simulink model "team_model_v1.2"  (R2022a)
settings: Solver=VariableStepAuto  StartTime=0.0  StopTime=10.0  RelTol=1e-3
undefined symbols (not defined in the file): dfilt, DiscIntNeverNeededParam, sigbuilder_block
libraries: visionsources x8, simulink x6, dsparch4 x5, dspvision x3, audioeffects x2, dspsnks4 x1, commanapbnd3 x1, commsynccomp2 x1
settings Model: Creator=Yogesh  LastModifiedBy=loges

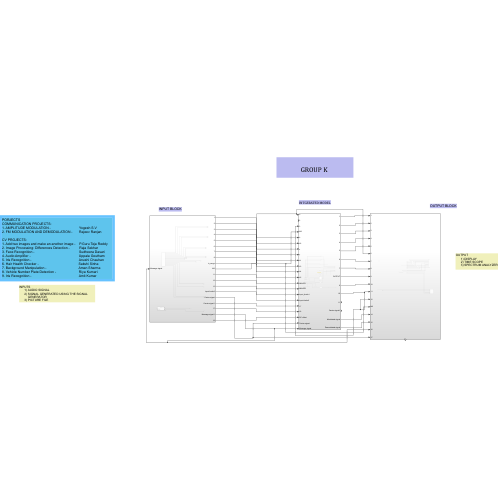
[thumbnail: Simulink's stored preview of the top-level diagram]
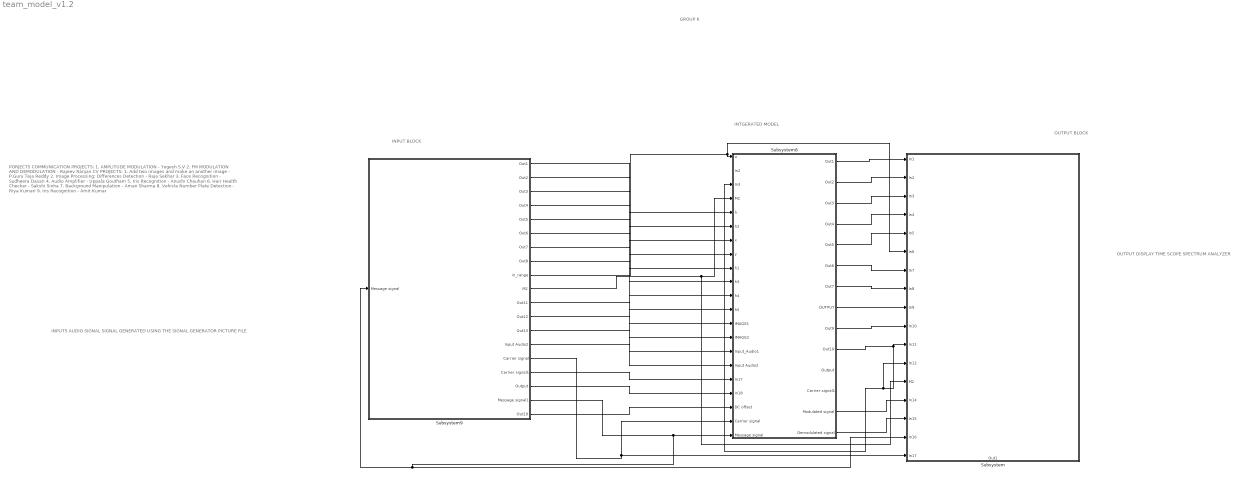
== system team_model_v1.2 ==
  note: OUTPUT
      | DISPLAY
      | TIME SCOPE
      | SPECTRUM ANALYZER
  note: INPUTS
      | AUDIO SIGNAL
      | SIGNAL GENERATED USING THE SIGNAL GENERATOR
      | PICTURE FILE
  note: PORJECTS
      | COMMUNICATION PROJECTS:
      | 1. AMPLITUDE MODULATION - Yogesh S.V
      | 2. FM MODULATION AND DEMODULATION - Rajeev Ranjan
      |
      | CV PROJECTS:
      | 1. Add two images and make an another image - P.Guru Teja Reddy
      | 2. Image Processing: Differences Detection - Raja Sekhar
      | 3. Face Recognition - Sudheera Dasari
      | 4. Audio Amplifier - Uppala Goutham
      | 5. Iris Recognition - Anushi Chauhan
      | 6. Hair Health Checker - Sakshi Sinha
      | 7. Background Manipulation - Aman Sharma
      | 8. Vehicle Number Plate Detection - Riya Kumari
      | 9. Iris Recognition - Amit Kumar
  note: GROUP K
  note: OUTPUT BLOCK
  note: INPUT BLOCK
  note: INTGERATED MODEL
  Subsystem : Subsystem
      settings: PortSchema="{\"entries\":[{\"content\":{\"sides\":[{\"content\":{\"connectorIds\":[\"In1\",\"In2\",\"In3\",\"In4\",\"In5\",\"In6\",\"In7\",\"In8\",\"In9\",\"In10\",\"In11\",\"In12\",\"In13\",\"In14\",\"In15\",\"In16\",\"In17\"]},\"type\":\"ConnectorPlacement.EquallySpacedRectSide\",\"uuid\":\"30eb3b3b-e642-47c5-bd95-9ad21aad3d43\"},{\"content\":{\"connectorIds\":[],\"side\":\"RIGHT\"},\"type\":\"ConnectorPlacement.EquallySpacedRectSide\",\"uuid\":\"7c869e27-b9a3-4d84-b0f1-035dc5e7d885\"},{\"content\":{\"connectorIds\":[],\"side\":\"TOP\"},\"type\":\"ConnectorPlacement.EquallySpacedRectSide\",\"uuid\":\"1cca7824-1698-4971-845e-a337e380de9b\"},{\"content\":{\"connectorIds\":[\"Out1\"],\"side\":\"BOTTOM\"},\"type\":\"ConnectorPlacement.EquallySpacedRectSide\",\"uuid\":\"e608f006-b2e8-4151-859e-ece5e69022af\"}]},\"type\":\"ConnectorPlacement.EquallySpacedConnector\",\"uuid\":\"a6df2039-72ad-42ba-adc3-335df7237120\"}],\"packageUris\":[\"http://schema.mathworks.com/mf0/Connector/R2020b\"],\"version\":\"1.0\"}"
  Subsystem8 : Subsystem
  Subsystem9 : Subsystem
  wires:
  Subsystem9/9(in_range) -> Subsystem8/1(u), Subsystem/6(In6)
  Subsystem9/10(M2) -> Subsystem/13(M2), Subsystem8/4(M2)
  Subsystem9/15(Carrier signal) -> Subsystem8/20(Carrier signal), Subsystem/17(In17)
  Subsystem9/18(Message signal1) -> Subsystem/16(In16), Subsystem9/1(Message signal), Subsystem8/21(Message signal)
  Subsystem8/10(Out10) -> Subsystem8/3(In3), Subsystem/12(In12), Subsystem/11(In11)
  Subsystem9/1(Out1) -> Subsystem8/5(h)
  Subsystem9/2(Out2) -> Subsystem8/6(h2)
  Subsystem9/3(Out3) -> Subsystem8/7(x)
  Subsystem9/4(Out4) -> Subsystem8/8(y)
  Subsystem9/5(Out5) -> Subsystem8/9(h1)
  Subsystem9/6(Out6) -> Subsystem8/10(h3)
  Subsystem9/7(Out7) -> Subsystem8/11(h4)
  Subsystem9/8(Out8) -> Subsystem8/12(h5)
  Subsystem9/11(Out11) -> Subsystem8/13(IMAGE1)
  Subsystem9/12(Out12) -> Subsystem8/14(IMAGE2)
  Subsystem9/13(Out13) -> Subsystem8/15(Input_Audio1)
  Subsystem9/14(Input Audio2) -> Subsystem8/16(Input Audio2)
  Subsystem9/16(Carrier signal1) -> Subsystem8/17(In17)
  Subsystem9/17(Output) -> Subsystem8/18(In18)
  Subsystem9/19(Out19) -> Subsystem8/19(DC offset)
  Subsystem8/1(Out1) -> Subsystem/1(In1)
  Subsystem8/2(Out2) -> Subsystem/2(In2)
  Subsystem8/3(Out3) -> Subsystem/3(In3)
  Subsystem8/4(Out4) -> Subsystem/4(In4)
  Subsystem8/5(Out5) -> Subsystem/5(In5)
  Subsystem8/6(Out6) -> Subsystem/7(In7)
  Subsystem8/7(Out7) -> Subsystem/8(In8)
  Subsystem8/8(OUTPUT) -> Subsystem/9(In9)
  Subsystem8/9(Out9) -> Subsystem/10(In10)
  Subsystem8/13(Modulated signal) -> Subsystem/14(In14)
  Subsystem8/14(Demodulated signal) -> Subsystem/15(In15)

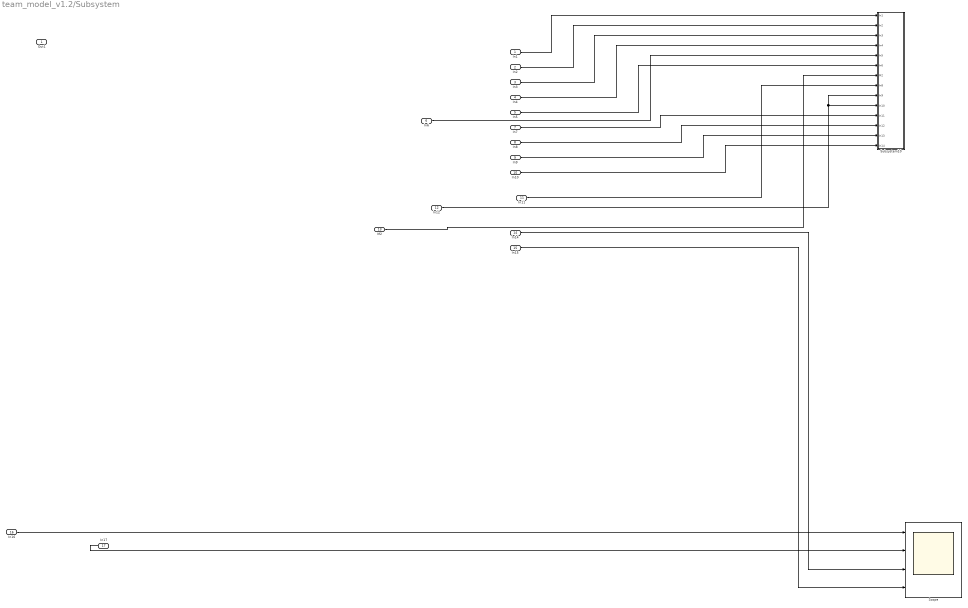
== system team_model_v1.2/Subsystem ==
  In1 : Inport
  In2 : Inport  Port=2
  In3 : Inport  Port=3
  In4 : Inport  Port=4
  In5 : Inport  Port=5
  In6 : Inport  Port=6
  In7 : Inport  Port=7
  In8 : Inport  Port=8
  In9 : Inport  Port=9
  In10 : Inport  Port=10
  In11 : Inport  Port=11
  In12 : Inport  Port=12
  M2 : Inport  Port=13
  In14 : Inport  Port=14
  In15 : Inport  Port=15
  In16 : Inport  Port=16
  In17 : Inport  Port=17
  Scope : Scope  NumInputPorts=4
  Subsystem10 : Subsystem
  Out1 : Outport
  wires:
  In16/1 -> Scope/1
  In12/1 -> Subsystem10/9(In9), Subsystem10/10(In10)
  In4/1 -> Subsystem10/4(In4)
  In10/1 -> Subsystem10/14(In14)
  In3/1 -> Subsystem10/3(In3)
  In11/1 -> Subsystem10/8(In8)
  In5/1 -> Subsystem10/6(In6)
  In2/1 -> Subsystem10/2(In2)
  In1/1 -> Subsystem10/1(In1)
  In6/1 -> Subsystem10/5(In5)
  In8/1 -> Subsystem10/12(In12)
  In7/1 -> Subsystem10/11(In11)
  In9/1 -> Subsystem10/13(In13)
  M2/1 -> Subsystem10/7(M2)
  In14/1 -> Scope/3
  In17/1 -> Scope/2
  In15/1 -> Scope/4

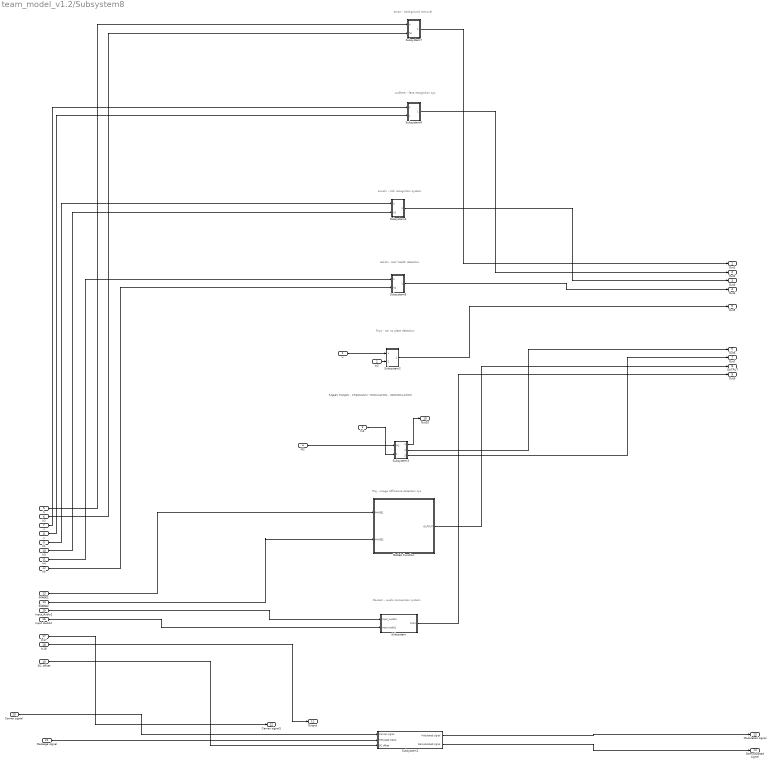
== system team_model_v1.2/Subsystem8 ==
  note: sudhera - face recognition sys
  note: anushi - irish recognition system
  note: sakshi - Hair health detection
  note: Riya - car no plate detection
  note: Raj - image difference detection sys
  note: Goutam - audio comaprison system
  note: RAJEEV RANJAN - FREQUENCY MODULATION - DEMODULATION
  note: Aman - background removal
  u : Inport
  In2 : Inport  Port=2
  In3 : Inport  Port=3
  M2 : Inport  Port=4
  h : Inport  Port=5
  h2 : Inport  Port=6
  x : Inport  Port=7
  y : Inport  Port=8
  h1 : Inport  Port=9
  h3 : Inport  Port=10
  h4 : Inport  Port=11
  h5 : Inport  Port=12
  IMAGE1 : Inport  Port=13
  IMAGE2 : Inport  Port=14
  Input_Audio1 : Inport  Port=15
  Input Audio2 : Inport  Port=16
  In17 : Inport  Port=17
  In18 : Inport  Port=18
  DC offset : Inport  Port=19
  Carrier signal : Inport  Port=20
  Message signal : Inport  Port=21
  Matlab Function : Subsystem
  Subsystem : Subsystem
  Subsystem1 : Subsystem
  Subsystem2 : Subsystem
  Subsystem3 : Subsystem
  Subsystem4 : Subsystem
  Subsystem5 : Subsystem
  Subsystem6 : Subsystem
  Subsystem7 : Subsystem
  Out1 : Outport
  Out2 : Outport  Port=2
  Out3 : Outport  Port=3
  Out4 : Outport  Port=4
  Out5 : Outport  Port=5
  Out6 : Outport  Port=6
  Out7 : Outport  Port=7
  OUTPUT : Outport  Port=8
  Out9 : Outport  Port=9
  Out10 : Outport  Port=10
  Output : Outport  Port=11
  Carrier signal1 : Outport  Port=12
  Modulated signal : Outport  Port=13
  Demodulated signal : Outport  Port=14
  wires:
  M2/1 -> Subsystem3/1(M2)
  Subsystem6/1(Out1) -> Out2/1
  Subsystem2/1(Out1) -> Out5/1
  y/1 -> Subsystem6/2(y)
  Subsystem3/2(Out2) -> Out6/1
  Subsystem7/1(Out1) -> Out1/1
  Subsystem3/3(Out3) -> Out7/1
  Subsystem5/1(Out1) -> Out4/1
  h3/1 -> Subsystem4/2(h2)
  Subsystem4/1(Out1) -> Out3/1
  u/1 -> Subsystem2/1(u)
  Matlab Function/1(OUTPUT) -> OUTPUT/1
  Subsystem/1(Out1) -> Out9/1
  h/1 -> Subsystem7/1(h)
  h2/1 -> Subsystem7/2(h2)
  x/1 -> Subsystem6/1(x)
  IMAGE2/1 -> Matlab Function/2(IMAGE2)
  Input_Audio1/1 -> Subsystem/1(Input_Audio1)
  h4/1 -> Subsystem5/1(h)
  In17/1 -> Carrier signal1/1
  Subsystem1/2(Demodulated signal) -> Demodulated signal/1
  IMAGE1/1 -> Matlab Function/1(IMAGE1)
  h1/1 -> Subsystem4/1(h)
  h5/1 -> Subsystem5/2(h2)
  In2/1 -> Subsystem2/2(In2)
  DC offset/1 -> Subsystem1/3(DC offset)
  In18/1 -> Output/1
  Input Audio2/1 -> Subsystem/2(Input Audio2)
  Message signal/1 -> Subsystem1/2(Message signal)
  Subsystem1/1(Modulated signal) -> Modulated signal/1
  Carrier signal/1 -> Subsystem1/1(Carrier signal)
  Subsystem3/1(Out1) -> Out10/1
  In3/1 -> Subsystem3/2(In2)

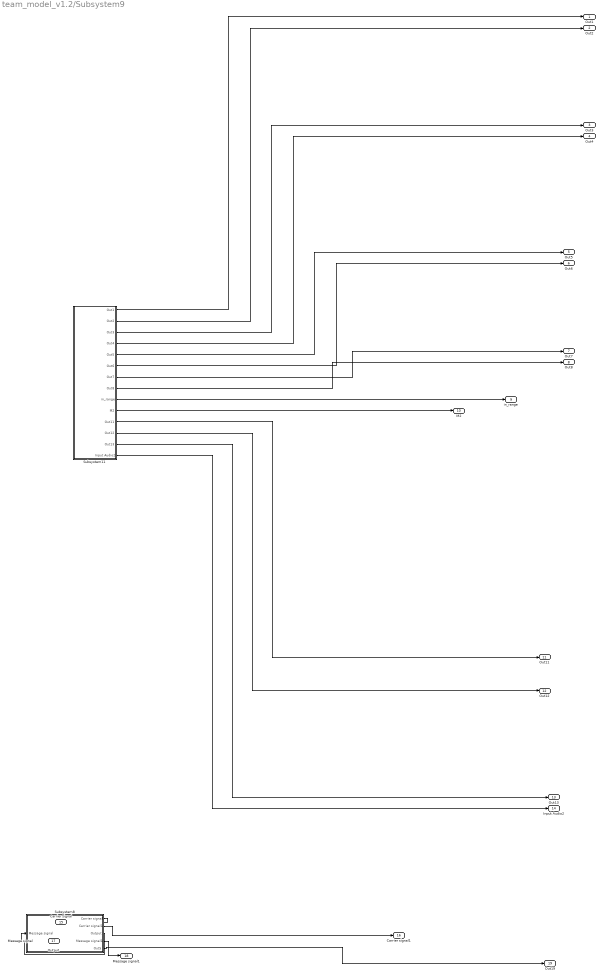
== system team_model_v1.2/Subsystem9 ==
  Message signal : Inport
  Subsystem11 : Subsystem
  Subsystem8 : Subsystem
  Out1 : Outport
  Out2 : Outport  Port=2
  Out3 : Outport  Port=3
  Out4 : Outport  Port=4
  Out5 : Outport  Port=5
  Out6 : Outport  Port=6
  Out7 : Outport  Port=7
  Out8 : Outport  Port=8
  in_range : Outport  Port=9
  M2 : Outport  Port=10
  Out11 : Outport  Port=11
  Out12 : Outport  Port=12
  Out13 : Outport  Port=13
  Input Audio2 : Outport  Port=14
  Carrier signal : Outport  Port=15
  Carrier signal1 : Outport  Port=16
  Output : Outport  Port=17
  Message signal1 : Outport  Port=18
  Out19 : Outport  Port=19
  wires:
  Subsystem8/5(Out5) -> Out19/1
  Subsystem8/3(Output) -> Output/1
  Subsystem8/1(Carrier signal) -> Carrier signal/1
  Subsystem11/2(Out2) -> Out2/1
  Message signal/1 -> Subsystem8/1(Message signal)
  Subsystem8/4(Message signal1) -> Message signal1/1
  Subsystem11/1(Out1) -> Out1/1
  Subsystem8/2(Carrier signal1) -> Carrier signal1/1
  Subsystem11/3(Out3) -> Out3/1
  Subsystem11/5(Out5) -> Out5/1
  Subsystem11/4(Out4) -> Out4/1
  Subsystem11/12(Out12) -> Out12/1
  Subsystem11/13(Out13) -> Out13/1
  Subsystem11/10(M2) -> M2/1
  Subsystem11/9(in_range) -> in_range/1
  Subsystem11/6(Out6) -> Out6/1
  Subsystem11/7(Out7) -> Out7/1
  Subsystem11/11(Out11) -> Out11/1
  Subsystem11/8(Out8) -> Out8/1
  Subsystem11/14(Input Audio2) -> Input Audio2/1

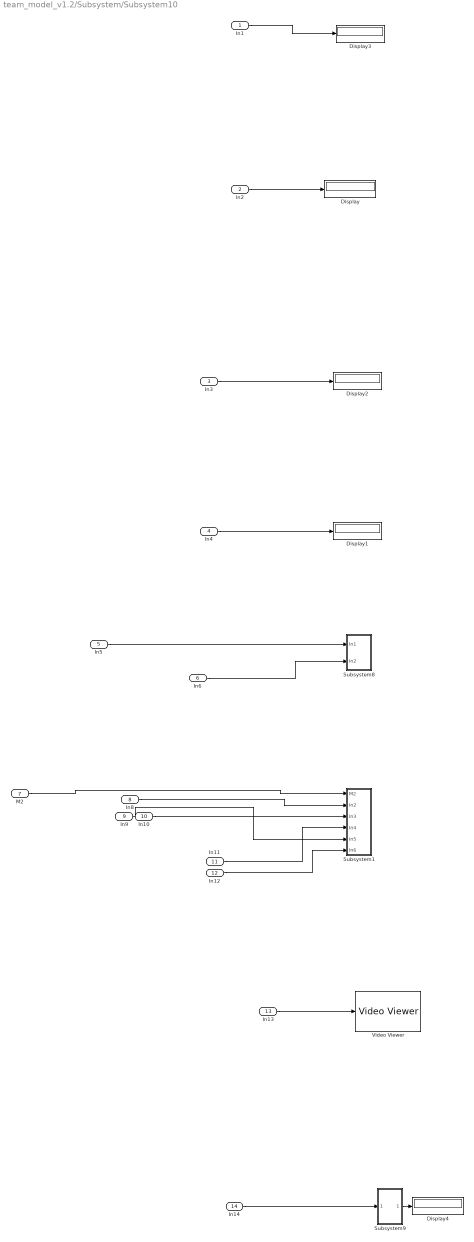
== system team_model_v1.2/Subsystem/Subsystem10 ==
  In1 : Inport
  In2 : Inport  Port=2
  In3 : Inport  Port=3
  In4 : Inport  Port=4
  In5 : Inport  Port=5
  In6 : Inport  Port=6
  M2 : Inport  Port=7
  In8 : Inport  Port=8
  In9 : Inport  Port=9
  In10 : Inport  Port=10
  In11 : Inport  Port=11
  In12 : Inport  Port=12
  In13 : Inport  Port=13
  In14 : Inport  Port=14
  Display{,1..4} (5 alike) : Display
  Subsystem1 : Subsystem
  Subsystem8 : Subsystem
  Subsystem9 : Subsystem
  Video Viewer : VideoViewer  FigPos=[1376 392 357 191]
  wires:
  In3/1 -> Display2/1
  In8/1 -> Subsystem1/2(In2)
  In13/1 -> Video Viewer/1
  In14/1 -> Subsystem9/1(In1)
  In9/1 -> Subsystem1/5(In5)
  In10/1 -> Subsystem1/3(In3)
  In1/1 -> Display3/1
  Subsystem9/1(Out1) -> Display4/1
  In4/1 -> Display1/1
  In2/1 -> Display/1
  In5/1 -> Subsystem8/1(In1)
  In6/1 -> Subsystem8/2(In2)
  In11/1 -> Subsystem1/4(In4)
  M2/1 -> Subsystem1/1(M2)
  In12/1 -> Subsystem1/6(In6)

== system team_model_v1.2/Subsystem8/Matlab Function ==
  IMAGE1 : Inport
  IMAGE2 : Inport  Port=2
  MATLAB Function : MATLAB Function  TreatAsAtomicUnit=on
  OUTPUT : Outport
  wires:
  IMAGE2/1 -> MATLAB Function/2(y)
  IMAGE1/1 -> MATLAB Function/1(x)
  MATLAB Function/1(z) -> OUTPUT/1

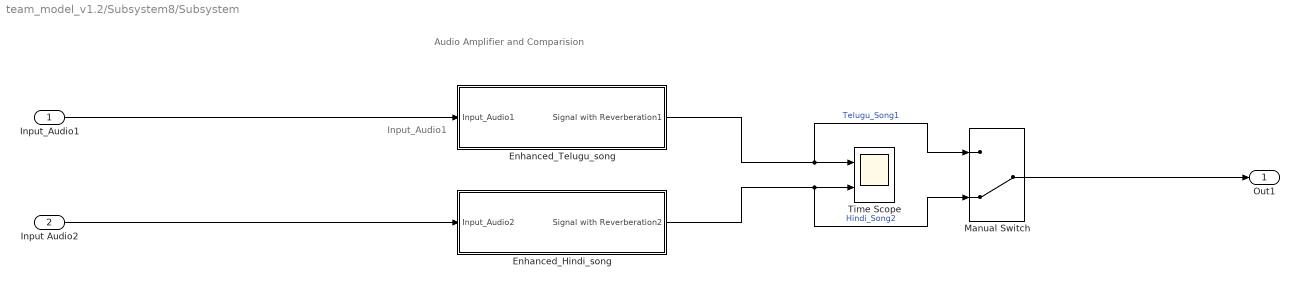
== system team_model_v1.2/Subsystem8/Subsystem ==
  note: Audio Amplifier and Comparision
  note: Input_Audio1
  Input_Audio1 : Inport
  Input Audio2 : Inport  Port=2
  " Manual Switch" : ManualSwitch  CurrentSetting=0
  Enhanced_Hindi_song : Subsystem
  Enhanced_Telugu_song : Subsystem
  Time Scope : Scope  NumInputPorts=2
  Out1 : Outport
  wires:
  " Manual Switch"/1 -> Out1/1
  Enhanced_Hindi_song/1(Signal with Reverberation2) -> " Manual Switch"/2, Time Scope/2  "Hindi_Song2"
  Enhanced_Telugu_song/1(Signal with Reverberation1) -> " Manual Switch"/1, Time Scope/1  "Telugu_Song1"
  Input Audio2/1 -> Enhanced_Hindi_song/1(Input_Audio2)
  Input_Audio1/1 -> Enhanced_Telugu_song/1(Input_Audio1)

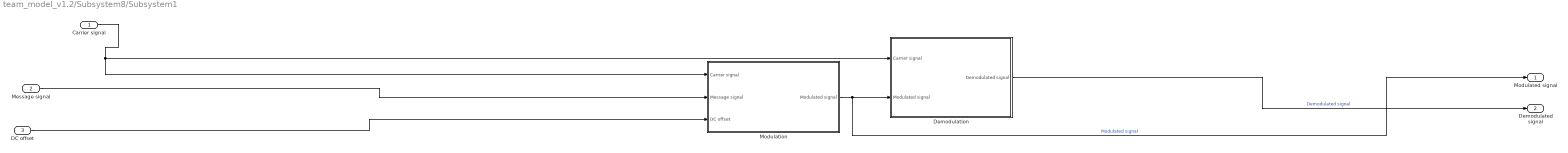
== system team_model_v1.2/Subsystem8/Subsystem1 ==
  Carrier signal : Inport
  Message signal : Inport  Port=2
  DC offset : Inport  Port=3
  Demodulation : Subsystem
  Modulation : Subsystem
  Modulated signal : Outport
  Demodulated signal : Outport  Port=2
  wires:
  Message signal/1 -> Modulation/2(Message signal)
  Modulation/1(Modulated signal) -> Modulated signal/1, Demodulation/2(Modulated signal)  "Modulated signal"
  DC offset/1 -> Modulation/3(DC offset)
  Carrier signal/1 -> Demodulation/1(Carrier signal), Modulation/1(Carrier signal)
  Demodulation/1(Demodulated signal) -> Demodulated signal/1  "Demodulated signal"

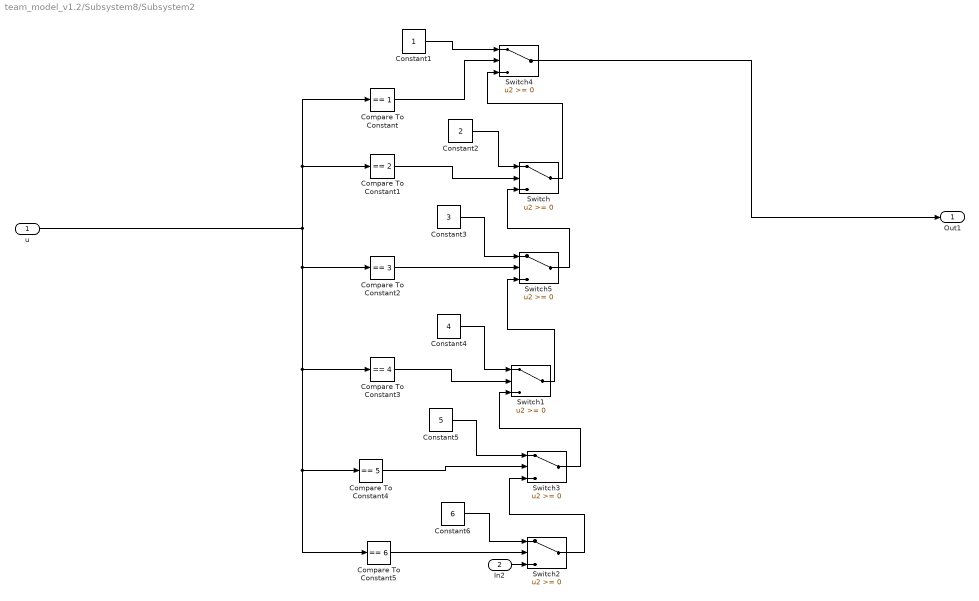
== system team_model_v1.2/Subsystem8/Subsystem2 ==
  u : Inport
  In2 : Inport  Port=2
  Compare To Constant : simulink/Logic and Bit Operations/Compare To Constant  relop===  const=1  OutDataTypeStr=boolean
  Compare To Constant1 : simulink/Logic and Bit Operations/Compare To Constant  relop===  const=2  OutDataTypeStr=boolean
  Compare To Constant2 : simulink/Logic and Bit Operations/Compare To Constant  relop===  const=3  OutDataTypeStr=boolean
  Compare To Constant3 : simulink/Logic and Bit Operations/Compare To Constant  relop===  const=4  OutDataTypeStr=boolean
  Compare To Constant4 : simulink/Logic and Bit Operations/Compare To Constant  relop===  const=5  OutDataTypeStr=boolean
  Compare To Constant5 : simulink/Logic and Bit Operations/Compare To Constant  relop===  const=6  OutDataTypeStr=boolean
  Constant1 : Constant
  Constant2 : Constant  Value=2
  Constant3 : Constant  Value=3
  Constant4 : Constant  Value=4
  Constant5 : Constant  Value=5
  Constant6 : Constant  Value=6
  Switch{,1..5} (6 alike) : Switch  SaturateOnIntegerOverflow=off  InputSameDT=off
  Out1 : Outport
  wires:
  Compare To Constant3/1 -> Switch1/2
  Compare To Constant/1 -> Switch4/2
  Switch1/1 -> Switch5/3
  Compare To Constant2/1 -> Switch5/2
  Switch2/1 -> Switch3/3
  u/1 -> Compare To Constant5/1, Compare To Constant4/1, Compare To Constant3/1, Compare To Constant2/1, Compare To Constant/1, Compare To Constant1/1
  Switch4/1 -> Out1/1
  Compare To Constant4/1 -> Switch3/2
  Compare To Constant5/1 -> Switch2/2
  Compare To Constant1/1 -> Switch/2
  Switch3/1 -> Switch1/3
  Switch5/1 -> Switch/3
  Switch/1 -> Switch4/3
  Constant1/1 -> Switch4/1
  Constant2/1 -> Switch/1
  Constant4/1 -> Switch1/1
  Constant3/1 -> Switch5/1
  Constant5/1 -> Switch3/1
  Constant6/1 -> Switch2/1
  In2/1 -> Switch2/3

== system team_model_v1.2/Subsystem8/Subsystem3 ==
  M2 : Inport
  In2 : Inport  Port=2
  "Subsystem(Indirect FM) " : Subsystem
  Subsystem2 : Subsystem
  Out1 : Outport
  Out2 : Outport  Port=2
  Out3 : Outport  Port=3
  wires:
  Subsystem2/1(Out1) -> Out2/1
  In2/1 -> Subsystem2/1(In1)
  Subsystem2/2(Out2) -> Out3/1
  M2/1 -> "Subsystem(Indirect FM) "/1(In1)
  "Subsystem(Indirect FM) "/1(Out1) -> Out1/1

== system team_model_v1.2/Subsystem8/Subsystem4 ==
  h : Inport
  h2 : Inport  Port=2
  MATLAB Function : MATLAB Function  TreatAsAtomicUnit=on
  MATLAB Function1 : MATLAB Function  TreatAsAtomicUnit=on
  Subsystem4 : Subsystem
  Out1 : Outport
  wires:
  MATLAB Function/1(y) -> Subsystem4/1(y)
  MATLAB Function1/1(y) -> Subsystem4/2(In2)
  h2/1 -> MATLAB Function1/1(h2)
  h/1 -> MATLAB Function/1(h)
  Subsystem4/1(Out1) -> Out1/1

== system team_model_v1.2/Subsystem8/Subsystem5 ==
  h : Inport
  h2 : Inport  Port=2
  MATLAB Function : MATLAB Function  TreatAsAtomicUnit=on
  MATLAB Function1 : MATLAB Function  TreatAsAtomicUnit=on
  Subsystem4 : Subsystem
  Out1 : Outport
  wires:
  MATLAB Function/1(y) -> Subsystem4/1(y)
  MATLAB Function1/1(y) -> Subsystem4/2(In2)
  h2/1 -> MATLAB Function1/1(h2)
  h/1 -> MATLAB Function/1(h)
  Subsystem4/1(Out1) -> Out1/1

== system team_model_v1.2/Subsystem8/Subsystem6 ==
  x : Inport
  y : Inport  Port=2
  MATLAB Function : MATLAB Function  TreatAsAtomicUnit=on
  String Constant : StringConstant  String="\"Same\""
  String Constant1 : StringConstant  String="\"Different\""
  Switch : Switch  Criteria=u2 ~= 0  SaturateOnIntegerOverflow=off  InputSameDT=off
  Out1 : Outport
  wires:
  Switch/1 -> Out1/1
  String Constant1/1 -> Switch/1
  String Constant/1 -> Switch/3
  MATLAB Function/1(z) -> Switch/2
  y/1 -> MATLAB Function/2(y)
  x/1 -> MATLAB Function/1(x)

== system team_model_v1.2/Subsystem8/Subsystem7 ==
  h : Inport
  h2 : Inport  Port=2
  MATLAB Function : MATLAB Function  TreatAsAtomicUnit=on
  MATLAB Function1 : MATLAB Function  TreatAsAtomicUnit=on
  Subsystem4 : Subsystem
  Out1 : Outport
  wires:
  MATLAB Function/1(y) -> Subsystem4/1(y)
  MATLAB Function1/1(y) -> Subsystem4/2(In2)
  h2/1 -> MATLAB Function1/1(h2)
  h/1 -> MATLAB Function/1(h)
  Subsystem4/1(Out1) -> Out1/1

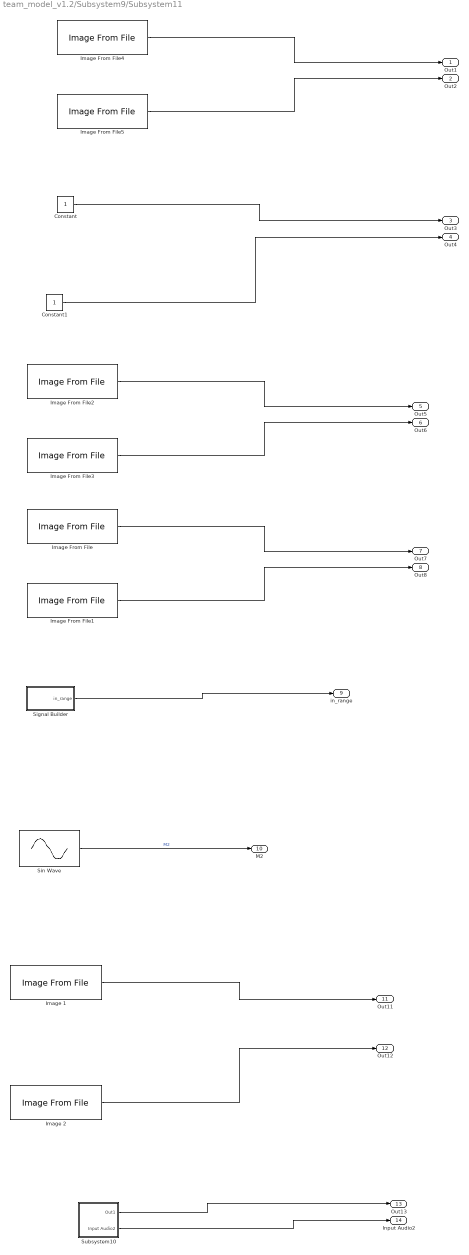
== system team_model_v1.2/Subsystem9/Subsystem11 ==
  Constant : Constant
  Constant1 : Constant
  Image 1 : visionsources/Image From File  Tag=vipblks_nd  FileName=D:\Users\RAJSEKHAR\Downloads\red2.jpg  Ts=inf  imagePorts=One multidimensional signal  OutPortLabels=R|G|B  ImageDataType=Inherit from input image  sdImageDataType=uint(8)  Signed=on  WordLength=16  FractionLengthMode=User-defined  FractionLength=15
  Image 2 : visionsources/Image From File  Tag=vipblks_nd  FileName=D:\Users\RAJSEKHAR\Downloads\tr5.jpg  Ts=inf  imagePorts=One multidimensional signal  OutPortLabels=R|G|B  ImageDataType=Inherit from input image  sdImageDataType=uint(8)  Signed=on  WordLength=16  FractionLengthMode=User-defined  FractionLength=15
  Image From File : visionsources/Image From File  Tag=vipblks_nd  FileName=C:\Users\LENOVO\OneDrive\Documents\L&T\MBD MATLAB\hair22.jpg  Ts=inf  imagePorts=One multidimensional signal  OutPortLabels=R|G|B  ImageDataType=Inherit from input image  sdImageDataType=uint(8)  Signed=on  WordLength=16  FractionLengthMode=User-defined  FractionLength=15
  Image From File1 : visionsources/Image From File  Tag=vipblks_nd  FileName=C:\Users\LENOVO\OneDrive\Documents\L&T\MBD MATLAB\hair21.jpg  Ts=inf  imagePorts=One multidimensional signal  OutPortLabels=R|G|B  ImageDataType=Inherit from input image  sdImageDataType=uint(8)  Signed=on  WordLength=16  FractionLengthMode=User-defined  FractionLength=15
  Image From File2 : visionsources/Image From File  Tag=vipblks_nd  FileName=C:\Users\LENOVO\OneDrive\Documents\L&T\MBD MATLAB\hair22.jpg  Ts=inf  imagePorts=One multidimensional signal  OutPortLabels=R|G|B  ImageDataType=Inherit from input image  sdImageDataType=uint(8)  Signed=on  WordLength=16  FractionLengthMode=User-defined  FractionLength=15
  Image From File3 : visionsources/Image From File  Tag=vipblks_nd  FileName=C:\Users\LENOVO\OneDrive\Documents\L&T\MBD MATLAB\hair21.jpg  Ts=inf  imagePorts=One multidimensional signal  OutPortLabels=R|G|B  ImageDataType=Inherit from input image  sdImageDataType=uint(8)  Signed=on  WordLength=16  FractionLengthMode=User-defined  FractionLength=15
  Image From File4 : visionsources/Image From File  Tag=vipblks_nd  FileName=C:\Users\LENOVO\OneDrive\Documents\L&T\MBD MATLAB\hair22.jpg  Ts=inf  imagePorts=One multidimensional signal  OutPortLabels=R|G|B  ImageDataType=Inherit from input image  sdImageDataType=uint(8)  Signed=on  WordLength=16  FractionLengthMode=User-defined  FractionLength=15
  Image From File5 : visionsources/Image From File  Tag=vipblks_nd  FileName=C:\Users\LENOVO\OneDrive\Documents\L&T\MBD MATLAB\hair21.jpg  Ts=inf  imagePorts=One multidimensional signal  OutPortLabels=R|G|B  ImageDataType=Inherit from input image  sdImageDataType=uint(8)  Signed=on  WordLength=16  FractionLengthMode=User-defined  FractionLength=15
  Signal Builder : Subsystem  Tag=STV Subsys  LoadFcn=sigbuilder_block('load');  StartFcn=sigbuilder_block('start');  StopFcn=sigbuilder_block('stop');  ClipboardFcn=sigbuilder_block('clipboard');  mask(Sigbuilder block){tuvar=[0:10]}
      mask help: Simulink:masks:SigbuilderBlock_MD
      mask init:
      | if ~strcmp(get_param(bdroot(gcbh),'SimulationStatus'),'stopped') tuvar = sigbuilder_block('maskInit'); end
      settings: CopyFcn=sigbuilder_block('copy');  DeleteFcn=sigbuilder_block('delete');  ModelCloseFcn=sigbuilder_block('modelClose');  PreSaveFcn=sigbuilder_block('preSave');  PauseFcn=sigbuilder_block('pause');  ContinueFcn=sigbuilder_block('continue');  NameChangeFcn=sigbuilder_block('namechange');  OpenFcn=sigbuilder_block('open',[437.6 199.2 550.4 400 ]);  CloseFcn=sigbuilder_block('close');
      mask Display: plot(0, 0, 100, 100,[2, 2, 32, 32, 2], [68, 8, 8, 68, 68],[32, 2], [38, 38], [32, 19, 2],[53, 60, 44], [32, 17, 17, 2],[16, 16, 31, 31]);txt = getActiveGroup(gcbh);text(2, 100, txt,'verticalAlignment', 'top');
  Sin Wave : Sin  Frequency=4  SampleTime=1/1000
  Subsystem10 : Subsystem
  Out1 : Outport
  Out2 : Outport  Port=2
  Out3 : Outport  Port=3
  Out4 : Outport  Port=4
  Out5 : Outport  Port=5
  Out6 : Outport  Port=6
  Out7 : Outport  Port=7
  Out8 : Outport  Port=8
  in_range : Outport  Port=9
  M2 : Outport  Port=10
  Out11 : Outport  Port=11
  Out12 : Outport  Port=12
  Out13 : Outport  Port=13
  Input Audio2 : Outport  Port=14
  wires:
  Image From File/1 -> Out7/1
  Image From File4/1 -> Out1/1
  Image From File2/1 -> Out5/1
  Image 1/1 -> Out11/1
  Image From File1/1 -> Out8/1
  Image From File3/1 -> Out6/1
  Image From File5/1 -> Out2/1
  Image 2/1 -> Out12/1
  Signal Builder/1(in_range) -> in_range/1
  Constant1/1 -> Out4/1
  Sin Wave/1 -> M2/1  "M2"
  Subsystem10/1(Out1) -> Out13/1
  Subsystem10/2(Input Audio2) -> Input Audio2/1
  Constant/1 -> Out3/1

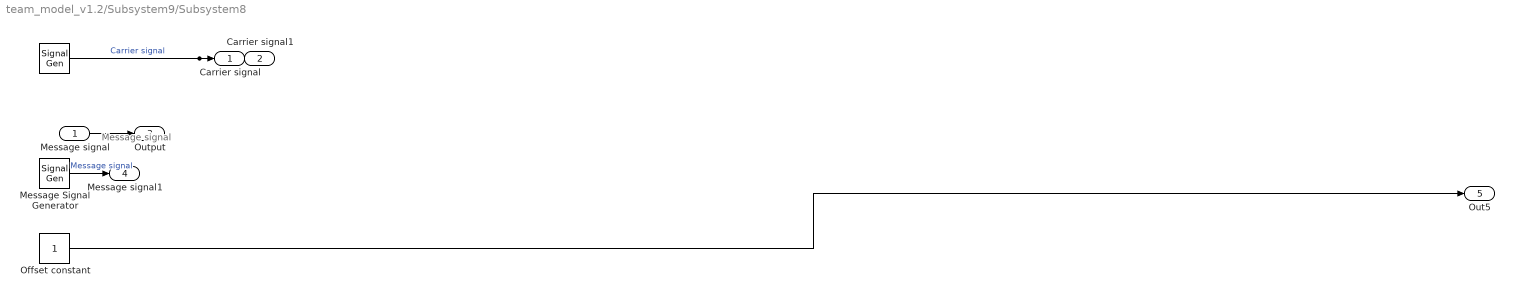
== system team_model_v1.2/Subsystem9/Subsystem8 ==
  note: Message signal
  Message signal : Inport
  " " : SignalGenerator  Amplitude=100  Frequency=2*pi*25  Units=rad/sec
  Message Signal Generator : SignalGenerator  Frequency=2*pi  Units=rad/sec
  Offset constant : Constant
  Carrier signal : Outport
  Carrier signal1 : Outport  Port=2
  Output : Outport  Port=3
  Message signal1 : Outport  Port=4
  Out5 : Outport  Port=5
  wires:
  Message signal/1 -> Output/1
  Offset constant/1 -> Out5/1
  " "/1 -> Carrier signal1/1, Carrier signal/1  "Carrier signal"
  Message Signal Generator/1 -> Message signal1/1  "Message signal"

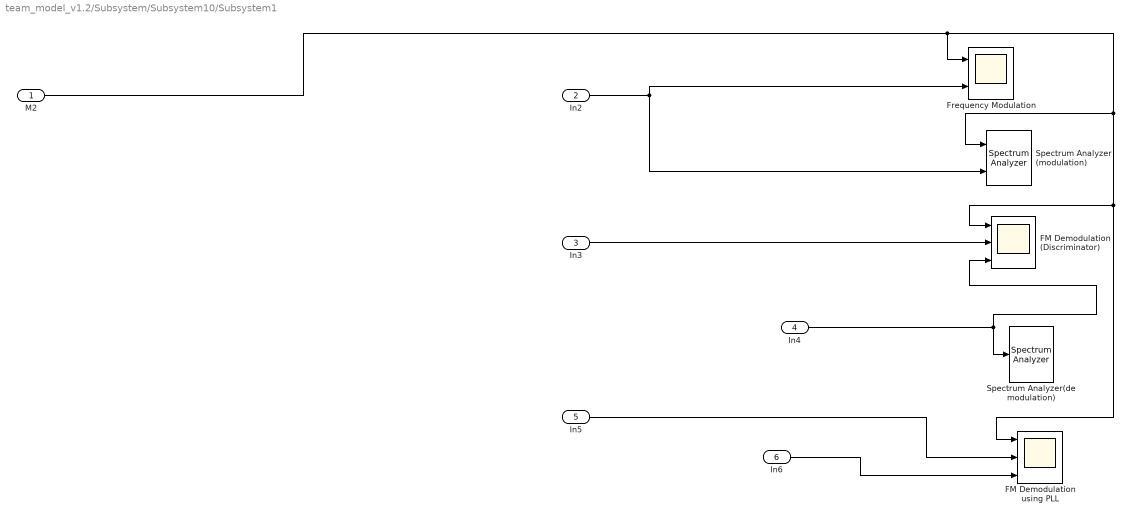
== system team_model_v1.2/Subsystem/Subsystem10/Subsystem1 ==
  M2 : Inport
  In2 : Inport  Port=2
  In3 : Inport  Port=3
  In4 : Inport  Port=4
  In5 : Inport  Port=5
  In6 : Inport  Port=6
  "                       FM Demodulation (Discriminator) " : Scope  NumInputPorts=3
  FM Demodulation using PLL : Scope  NumInputPorts=3
  "Frequency Modulation " : Scope  NumInputPorts=2
  "Spectrum Analyzer(demodulation) " : SpectrumAnalyzer
  Spectrum Analyzer (modulation) : SpectrumAnalyzer  NumInputPorts=2
  wires:
  M2/1 -> Spectrum Analyzer (modulation)/1, FM Demodulation using PLL/1, "                       FM Demodulation (Discriminator) "/1, "Frequency Modulation "/1
  In5/1 -> FM Demodulation using PLL/2
  In4/1 -> "                       FM Demodulation (Discriminator) "/3, "Spectrum Analyzer(demodulation) "/1
  In2/1 -> "Frequency Modulation "/2, Spectrum Analyzer (modulation)/2
  In6/1 -> FM Demodulation using PLL/3
  In3/1 -> "                       FM Demodulation (Discriminator) "/2

== system team_model_v1.2/Subsystem/Subsystem10/Subsystem8 ==
  In1 : Inport
  In2 : Inport  Port=2
  Display : Display
  Scope : Scope  NumInputPorts=2
  wires:
  In2/1 -> Scope/2, Display/1
  In1/1 -> Scope/1

== system team_model_v1.2/Subsystem/Subsystem10/Subsystem9 ==
  In1 : Inport
  " Audio file Recorder" : dspvision/To Multimedia File  outputFilename=E:\MathWorks\Project\audio_cut\output.wav  streamSelection=Audio only  videoCompressor=None (uncompressed)  audioCompressor=None (uncompressed)  imagePorts=Separate color signals  fileType=WAV  audioDatatype=16-bit integer  fourcc=RGB  videoQuality=75  mj2000CompFactor=10
  Audio Output : dspsnks4/Audio Device Writer  Driver=DirectSound  Device=Default  InheritSampleRate=on  SampleRate=44100  BitDepth=16-bit integer  BufferSize=4096  NumBuffers=10  DefaultOutputChannelMapping=on  OutputChannelMapping=1:2  OutputNumUnderrunSamples=off  DriverIdx=1  DeviceWarnFlag=''
  Out1 : Outport
  wires:
  In1/1 -> Audio Output/1, " Audio file Recorder"/1

== system team_model_v1.2/Subsystem8/Subsystem/Enhanced_Hindi_song ==
  Input_Audio2 : Inport
  "Filter " : Subsystem
  Reverberator2 : audioeffects/Reverberator  PreDelayPort=off  PreDelay=0.150  HighCutFrequencyPort=off  HighCutFrequency=20000  DiffusionPort=off  Diffusion=0.470  DecayFactorPort=off  DecayFactor=0.330  HighFrequencyDampingPort=off  HighFrequencyDamping=0.270  WetDryMixPort=off  WetDryMix=0.460  InheritSampleRate=on  SampleRate=44100  SimulateUsing=Interpreted execution
      settings: SourceProductBaseCode=AU
  Signal with Reverberation2 : Outport
  wires:
  "Filter "/1(Out1) -> Reverberator2/1  "filtered_Audio2"
  Input_Audio2/1 -> "Filter "/1(In1)
  Reverberator2/1 -> Signal with Reverberation2/1  "Signal with Reverberation 2"

== system team_model_v1.2/Subsystem8/Subsystem/Enhanced_Telugu_song ==
  Input_Audio1 : Inport
  "Filter " : Subsystem
  Reverberator2 : audioeffects/Reverberator  PreDelayPort=off  PreDelay=0.150  HighCutFrequencyPort=off  HighCutFrequency=20000  DiffusionPort=off  Diffusion=0.470  DecayFactorPort=off  DecayFactor=0.330  HighFrequencyDampingPort=off  HighFrequencyDamping=0.270  WetDryMixPort=off  WetDryMix=0.460  InheritSampleRate=on  SampleRate=44100  SimulateUsing=Interpreted execution
      settings: SourceProductBaseCode=AU
  Signal with Reverberation1 : Outport
  wires:
  "Filter "/1(Out1) -> Reverberator2/1  "filtered_Audio1"
  Input_Audio1/1 -> "Filter "/1(In1)
  Reverberator2/1 -> Signal with Reverberation1/1  "Signal with Reverberation 1"

== system team_model_v1.2/Subsystem8/Subsystem1/Demodulation ==
  note: Demodulation Subsystem
  Carrier signal : Inport
  Modulated signal : Inport  Port=2
  Demodulation : Product
  Transfer Fcn : TransferFcn  Numerator=[15]  Denominator=[1 15]
  Demodulated signal : Outport
  wires:
  Modulated signal/1 -> Demodulation/2
  Demodulation/1 -> Transfer Fcn/1
  Transfer Fcn/1 -> Demodulated signal/1  "Demodulated signal"
  Carrier signal/1 -> Demodulation/1

== system team_model_v1.2/Subsystem8/Subsystem1/Modulation ==
  note: Modulation
  Carrier signal : Inport
  Message signal : Inport  Port=2
  DC offset : Inport  Port=3
  Offset addition : Sum
  modulation1 : Product
  Modulated signal : Outport
  wires:
  modulation1/1 -> Modulated signal/1  "Modulated signal"
  Offset addition/1 -> modulation1/2
  Carrier signal/1 -> modulation1/1
  Message signal/1 -> Offset addition/1
  DC offset/1 -> Offset addition/2

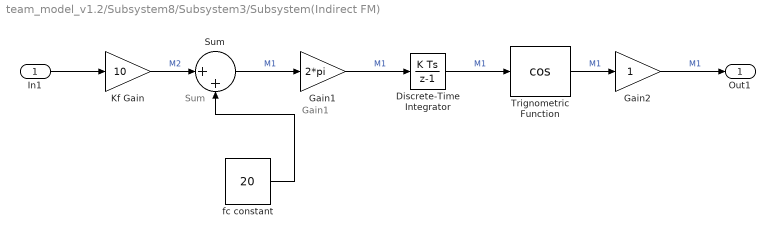
== system team_model_v1.2/Subsystem8/Subsystem3/Subsystem(Indirect FM)  ==
  note: Sum
  note: Gain1
  In1 : Inport
  "Discrete-Time Integrator " : DiscreteIntegrator  SampleTime=-1  ICPrevOutput=DiscIntNeverNeededParam  ICPrevScaledInput=DiscIntNeverNeededParam
  Gain1 : Gain  Gain=2*pi
  "Gain2 " : Gain
  Kf Gain : Gain  Gain=10
  Sum : Sum  Inputs=|++
  Trignometric Function : Trigonometry  Operator=cos
  fc constant : Constant  Value=20
  Out1 : Outport
  wires:
  Gain1/1 -> "Discrete-Time Integrator "/1  "M1"
  Sum/1 -> Gain1/1  "M1"
  Kf Gain/1 -> Sum/1  "M2"
  "Gain2 "/1 -> Out1/1  "M1"
  In1/1 -> Kf Gain/1
  "Discrete-Time Integrator "/1 -> Trignometric Function/1  "M1"
  Trignometric Function/1 -> "Gain2 "/1  "M1"
  fc constant/1 -> Sum/2

== system team_model_v1.2/Subsystem8/Subsystem3/Subsystem2 ==
  In1 : Inport
  "FM Demodulator Passband " : commanapbnd3/FM Demodulator Passband  Fc=20  Ph=0  Kc=10  Ho=200
      settings: SourceProductBaseCode=CM
  "Subsystem(Phase lock loop) " : Subsystem
  Out1 : Outport
  Out2 : Outport  Port=2
  wires:
  In1/1 -> "Subsystem(Phase lock loop) "/1(In1), "FM Demodulator Passband "/1
  "FM Demodulator Passband "/1 -> Out1/1
  "Subsystem(Phase lock loop) "/1(Out1) -> Out2/1

== system team_model_v1.2/Subsystem8/Subsystem4/Subsystem4 ==
  y : Inport
  In2 : Inport  Port=2
  MATLAB Function : MATLAB Function  TreatAsAtomicUnit=on
  String Constant : StringConstant  String="\"Not Healthy\""
  String Constant1 : StringConstant  String="\"Healthy\""
  Switch : Switch  Criteria=u2 > Threshold  SaturateOnIntegerOverflow=off  InputSameDT=off
  Out1 : Outport
  wires:
  y/1 -> MATLAB Function/1(h1)
  In2/1 -> MATLAB Function/2(h2)
  Switch/1 -> Out1/1
  String Constant/1 -> Switch/1
  String Constant1/1 -> Switch/3
  MATLAB Function/1(y) -> Switch/2

== system team_model_v1.2/Subsystem8/Subsystem5/Subsystem4 ==
  y : Inport
  In2 : Inport  Port=2
  MATLAB Function : MATLAB Function  TreatAsAtomicUnit=on
  String Constant : StringConstant  String="\"Not Healthy\""
  String Constant1 : StringConstant  String="\"Healthy\""
  Switch : Switch  Criteria=u2 > Threshold  SaturateOnIntegerOverflow=off  InputSameDT=off
  Out1 : Outport
  wires:
  y/1 -> MATLAB Function/1(h1)
  In2/1 -> MATLAB Function/2(h2)
  Switch/1 -> Out1/1
  String Constant/1 -> Switch/1
  String Constant1/1 -> Switch/3
  MATLAB Function/1(y) -> Switch/2

== system team_model_v1.2/Subsystem8/Subsystem7/Subsystem4 ==
  y : Inport
  In2 : Inport  Port=2
  MATLAB Function : MATLAB Function  TreatAsAtomicUnit=on
  String Constant : StringConstant  String="\"Not Healthy\""
  String Constant1 : StringConstant  String="\"Healthy\""
  Switch : Switch  Criteria=u2 > Threshold  SaturateOnIntegerOverflow=off  InputSameDT=off
  Out1 : Outport
  wires:
  y/1 -> MATLAB Function/1(h1)
  In2/1 -> MATLAB Function/2(h2)
  Switch/1 -> Out1/1
  String Constant/1 -> Switch/1
  String Constant1/1 -> Switch/3
  MATLAB Function/1(y) -> Switch/2

== system team_model_v1.2/Subsystem9/Subsystem11/Signal Builder ==
  Demux : Demux  Tag=STV Demux  Outputs=1
      settings: DisplayOption=none
  FromWs : FromWorkspace  Tag=STV FromWs  VariableName=tuvar
      SigBuilderData=|
      | common.afterFinalStr = 'Extrapolate'
      | common.sampleTime = 0
      | dataSet.timeRange = [1 9]
      | dataSet.name = 'Sheet1'
      | sbobj.Groups.Name = 'Sheet1'
      | sbobj.Groups.Signals.Name = 'in_range'
      | sbobj.Groups.Signals.XData = [1 2 3 4 5 6 7 8 9]
      | sbobj.Groups.Signals.YData = [0 1 1 0 0 1 1 0 0]
      | sbobj.Groups.TimeRange = [1 9]
  in_range : Outport  Tag=STV Outport
  wires:
  Demux/1 -> in_range/1
  FromWs/1 -> Demux/1

== system team_model_v1.2/Subsystem9/Subsystem11/Subsystem10 ==
  Hindi_Song : dspvision/From Multimedia File  inputFilename=E:\MathWorks\Project\audio_cut\Puspha\JaagoJaago Bakre (mp3cut.net).mp3  readRange=[1 Inf]  loop=on  numPlays=inf  outputStreams=Audio only  videoDataType=single  audioDataType=double  inheritSampleTime=on  userDefinedSampleTime=1/30  noAudioOutput=off  isIntensityVideo=off  fourcc=RGB  colorVideoFormat=Separate color signals  outputEOF=off  dataOrg=Column-major  audioFrameSize=1026  computeAudioFrameSize=off  outSamplingMode=Sample based
  Telugu_Song : dspvision/From Multimedia File  inputFilename=E:\MathWorks\Project\audio_cut\Puspha\Dakko Dakko Meka (mp3cut.net).mp3  readRange=[1 Inf]  loop=on  numPlays=inf  outputStreams=Audio only  videoDataType=single  audioDataType=double  inheritSampleTime=on  userDefinedSampleTime=1/30  noAudioOutput=off  isIntensityVideo=off  fourcc=RGB  colorVideoFormat=Separate color signals  outputEOF=off  dataOrg=Column-major  audioFrameSize=1026  computeAudioFrameSize=off  outSamplingMode=Sample based
  Out1 : Outport
  Input Audio2 : Outport  Port=2
  wires:
  Telugu_Song/1 -> Out1/1
  Hindi_Song/1 -> Input Audio2/1  "Input Audio2"

== system team_model_v1.2/Subsystem8/Subsystem/Enhanced_Hindi_song/Filter  ==
  In1 : Inport
  Biquad Filter : dsparch4/Biquad Filter  FilterSource=Dialog parameters  CoeffSource=Specify via dialog  FilterObject=dfilt.df2tsos([1 0.3 0.4],[1 0.1 0.2])  IIRFiltStruct=Direct form II transposed  BiQuadCoeffs=[1 0.3 0.4 1 0.1 0.2]  ScaleValues=1  IC=0  ICnum=0  ICden=0  a0Flag=Warning  optimizeScaleValues=on  ScaleValueMode=Specify via input port (g)  roundingMode=Floor  overflowMode=off  scaleValueFracLength=14  denProdOutputFracLength=30  denAccumFracLength=30  secondMemoryFracLength=15
  Biquad Filter1 : dsparch4/Biquad Filter  FilterSource=Dialog parameters  CoeffSource=Specify via dialog  FilterObject=dfilt.df2tsos([1 0.3 0.4],[1 0.1 0.2])  IIRFiltStruct=Direct form II transposed  BiQuadCoeffs=[1 0.3 0.4 1 0.1 0.2]  ScaleValues=1  IC=0  ICnum=0  ICden=0  a0Flag=Warning  optimizeScaleValues=on  ScaleValueMode=Specify via input port (g)  roundingMode=Floor  overflowMode=off  scaleValueFracLength=14  denProdOutputFracLength=30  denAccumFracLength=30  secondMemoryFracLength=15
  Out1 : Outport
  wires:
  In1/1 -> Biquad Filter/1
  Biquad Filter/1 -> Biquad Filter1/1
  Biquad Filter1/1 -> Out1/1

== system team_model_v1.2/Subsystem8/Subsystem/Enhanced_Telugu_song/Filter  ==
  In1 : Inport
  Biquad Filter : dsparch4/Biquad Filter  FilterSource=Dialog parameters  CoeffSource=Specify via dialog  FilterObject=dfilt.df2tsos([1 0.3 0.4],[1 0.1 0.2])  IIRFiltStruct=Direct form II transposed  BiQuadCoeffs=[1 0.3 0.4 1 0.1 0.2]  ScaleValues=1  IC=0  ICnum=0  ICden=0  a0Flag=Warning  optimizeScaleValues=on  ScaleValueMode=Specify via input port (g)  roundingMode=Floor  overflowMode=off  scaleValueFracLength=14  denProdOutputFracLength=30  denAccumFracLength=30  secondMemoryFracLength=15
  Biquad Filter1 : dsparch4/Biquad Filter  FilterSource=Dialog parameters  CoeffSource=Specify via dialog  FilterObject=dfilt.df2tsos([1 0.3 0.4],[1 0.1 0.2])  IIRFiltStruct=Direct form II transposed  BiQuadCoeffs=[1 0.3 0.4 1 0.1 0.2]  ScaleValues=1  IC=0  ICnum=0  ICden=0  a0Flag=Warning  optimizeScaleValues=on  ScaleValueMode=Specify via input port (g)  roundingMode=Floor  overflowMode=off  scaleValueFracLength=14  denProdOutputFracLength=30  denAccumFracLength=30  secondMemoryFracLength=15
  Out1 : Outport
  wires:
  In1/1 -> Biquad Filter/1
  Biquad Filter/1 -> Biquad Filter1/1
  Biquad Filter1/1 -> Out1/1

== system team_model_v1.2/Subsystem8/Subsystem3/Subsystem2/Subsystem(Phase lock loop)  ==
  In1 : Inport
  "Analog Filter Design " : dsparch4/Analog Filter Design  method=Butterworth  filttype=Lowpass  N=10  Wlo=2  Whi=80  Rp=2  Rs=40
  "Continuous-Time VCO " : commsynccomp2/Continuous-Time VCO  Ac=1  Fc=20  Kc=10/(2*pi)  Ph=pi/2
      settings: SourceProductBaseCode=CM
  "Gain3 " : Gain  Gain=10
  MatrixMultiply : Product  Multiplication=Matrix(*)
  Out1 : Outport
  wires:
  "Analog Filter Design "/1 -> "Continuous-Time VCO "/1, "Gain3 "/1
  "Continuous-Time VCO "/1 -> MatrixMultiply/2
  In1/1 -> MatrixMultiply/1
  MatrixMultiply/1 -> "Analog Filter Design "/1  "Const"
  "Gain3 "/1 -> Out1/1

== matlab function team_model_v1.2/Subsystem8/Subsystem5/MATLAB Function ==
  data: h input; y output
function y = fcn(h)
h = imread('hair22.jpg');
%imshow(h)
[count,x] = imhist(h);
sz = size(h);
R = h(:,:,1);
%imshow(R)

%to grayscale
red=h(:,:,1);
green=h(:,:,2);
blue=h(:,:,3);
image_gray = im2gray(h);
% figure (1),subplot (3,3,2), imshow(image_gray), title('grayscale');

%tobinary
level = graythresh(image_gray);
BW = imbinarize (image_gray,level);
% figure(1),subplot(3,3,3),imshow(BW), title('binary');

%closing
se = strel('disk',10);
afterclosing = imclose(BW,se);
% figure(1), subplot (3,3,4), imshow(afterclosing), title('closing');

%opening
afteropen = imopen(afterclosing,se);
% figure(1), subplot (3,3,5),imshow(afteropen), title('opening');


y = level;
end

== matlab function team_model_v1.2/Subsystem8/Subsystem5/MATLAB Function1 ==
  data: h2 input; y output
function y = fcn(h2)
h2 = imread('hair21.jpg');
%imshow(h2)
R2 = h2(:,:,1);
%imshow(R2)

%to grayscale
red2=h2(:,:,1);
green2=h2(:,:,2);
blue2=h2(:,:,3);
image_gray1 = im2gray(h2);
%figure (1),subplot (3,3,2), imshow(image_gray1), title('grayscale2');

%tobinary
level2 = graythresh(image_gray1);
BW2 = imbinarize (image_gray1,level2);
%figure(1),subplot(3,3,3),imshow(BW2), title('binary2');

%closing
se2 = strel('disk',10);
afterclosing2 = imclose(BW2,se2);
%figure(1), subplot (3,3,4), imshow(afterclosing2), title('closing2');

%opening
afteropen2 = imopen(afterclosing2 ,se2);
%figure(1), subplot (3,3,5),imshow(afteropen2), title('opening2');

y = level2;

== matlab function team_model_v1.2/Subsystem8/Subsystem5/Subsystem4/MATLAB Function ==
  data: h1 input; y output; h2 input
function y = fcn(h1, h2)
if(h1>h2)
    y=1;
else
    y=0;
end

end

== matlab function team_model_v1.2/Subsystem8/Subsystem4/MATLAB Function ==
  data: h input; y output
function y = fcn(h)
h = imread('hair22.jpg');
%imshow(h)
[count,x] = imhist(h);
sz = size(h);
R = h(:,:,1);
%imshow(R)

%to grayscale
red=h(:,:,1);
green=h(:,:,2);
blue=h(:,:,3);
image_gray = im2gray(h);
% figure (1),subplot (3,3,2), imshow(image_gray), title('grayscale');

%tobinary
level = graythresh(image_gray);
BW = imbinarize (image_gray,level);
% figure(1),subplot(3,3,3),imshow(BW), title('binary');

%closing
se = strel('disk',10);
afterclosing = imclose(BW,se);
% figure(1), subplot (3,3,4), imshow(afterclosing), title('closing');

%opening
afteropen = imopen(afterclosing,se);
% figure(1), subplot (3,3,5),imshow(afteropen), title('opening');


y = level;
end

== matlab function team_model_v1.2/Subsystem8/Subsystem4/MATLAB Function1 ==
  data: h2 input; y output
function y = fcn(h2)
h2 = imread('hair21.jpg');
%imshow(h2)
R2 = h2(:,:,1);
%imshow(R2)

%to grayscale
red2=h2(:,:,1);
green2=h2(:,:,2);
blue2=h2(:,:,3);
image_gray1 = im2gray(h2);
%figure (1),subplot (3,3,2), imshow(image_gray1), title('grayscale2');

%tobinary
level2 = graythresh(image_gray1);
BW2 = imbinarize (image_gray1,level2);
%figure(1),subplot(3,3,3),imshow(BW2), title('binary2');

%closing
se2 = strel('disk',10);
afterclosing2 = imclose(BW2,se2);
%figure(1), subplot (3,3,4), imshow(afterclosing2), title('closing2');

%opening
afteropen2 = imopen(afterclosing2 ,se2);
%figure(1), subplot (3,3,5),imshow(afteropen2), title('opening2');

y = level2;

== matlab function team_model_v1.2/Subsystem8/Subsystem4/Subsystem4/MATLAB Function ==
  data: h1 input; y output; h2 input
function y = fcn(h1, h2)
if(h1>h2)
    y=1;
else
    y=0;
end

end

== matlab function team_model_v1.2/Subsystem8/Subsystem6/MATLAB Function ==
  data: x input; z output; y input
function z = fcn(x,y)
g=size(x);
y=imresize(y,[g(1),g(2)]);
figure;
if(x==y)
    z=1;
else
    z=0;
end

== matlab function team_model_v1.2/Subsystem8/Subsystem7/MATLAB Function ==
  data: h input; y output
function y = fcn(h)
h = imread('hair22.jpg');
%imshow(h)
[count,x] = imhist(h);
sz = size(h);
R = h(:,:,1);
%imshow(R)

%to grayscale
red=h(:,:,1);
green=h(:,:,2);
blue=h(:,:,3);
image_gray = im2gray(h);
% figure (1),subplot (3,3,2), imshow(image_gray), title('grayscale');

%tobinary
level = graythresh(image_gray);
BW = imbinarize (image_gray,level);
% figure(1),subplot(3,3,3),imshow(BW), title('binary');

%closing
se = strel('disk',10);
afterclosing = imclose(BW,se);
% figure(1), subplot (3,3,4), imshow(afterclosing), title('closing');

%opening
afteropen = imopen(afterclosing,se);
% figure(1), subplot (3,3,5),imshow(afteropen), title('opening');


y = level;
end

== matlab function team_model_v1.2/Subsystem8/Subsystem7/MATLAB Function1 ==
  data: h2 input; y output
function y = fcn(h2)
h2 = imread('hair21.jpg');
%imshow(h2)
R2 = h2(:,:,1);
%imshow(R2)

%to grayscale
red2=h2(:,:,1);
green2=h2(:,:,2);
blue2=h2(:,:,3);
image_gray1 = im2gray(h2);
%figure (1),subplot (3,3,2), imshow(image_gray1), title('grayscale2');

%tobinary
level2 = graythresh(image_gray1);
BW2 = imbinarize (image_gray1,level2);
%figure(1),subplot(3,3,3),imshow(BW2), title('binary2');

%closing
se2 = strel('disk',10);
afterclosing2 = imclose(BW2,se2);
%figure(1), subplot (3,3,4), imshow(afterclosing2), title('closing2');

%opening
afteropen2 = imopen(afterclosing2 ,se2);
%figure(1), subplot (3,3,5),imshow(afteropen2), title('opening2');

y = level2;

== matlab function team_model_v1.2/Subsystem8/Matlab Function/MATLAB Function ==
  data: x input; z output; y input
function z = fcn(x, y)

%  clc
% clear
% close all
% warning off;
%  x=imread('D:\Users\RAJSEKHAR\Downloads\red2.jpg');
%  y=imread('D:\Users\RAJSEKHAR\Downloads\rect2.jpg');
g=size(x);
y=imresize(y,[g(1),g(2)]);
figure;
z=x-y;
pause(5);

== matlab function team_model_v1.2/Subsystem8/Subsystem7/Subsystem4/MATLAB Function ==
  data: h1 input; y output; h2 input
function y = fcn(h1, h2)
if(h1>h2)
    y=1;
else
    y=0;
end

end
